simulink library "AMKMotor"  (R2015a)
settings: Solver=ode45  StartTime=0.0  StopTime=10.0  RelTol=1e-3
undefined symbols (not defined in the file): Motor
libraries: driveline x1, simulink x1
settings Model: Creator=BRIAN  LastModifiedBy=BRIAN

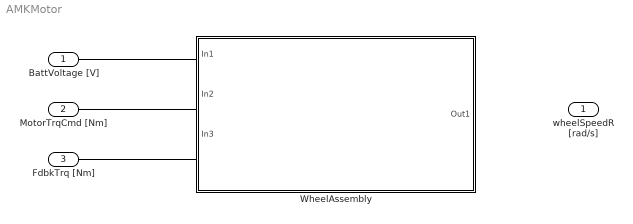
== system AMKMotor ==
  BattVoltage [V] : Inport
  MotorTrqCmd [Nm] : Inport  Port=2
  FdbkTrq [Nm] : Inport  Port=3
  WheelAssembly : Subsystem
  wheelSpeedR [rad/s] : Outport
  wires:
  BattVoltage [V]/1 -> ?
  MotorTrqCmd [Nm]/1 -> ?
  FdbkTrq [Nm]/1 -> ?
  ? -> wheelSpeedR [rad/s]/1

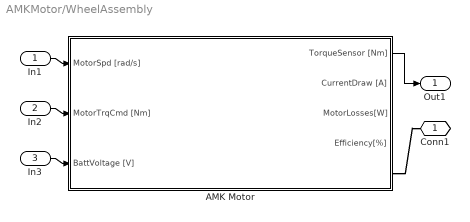
== system AMKMotor/WheelAssembly ==
  In1 : Inport
  In2 : Inport  Port=2
  In3 : Inport  Port=3
  AMK Motor : Subsystem
  Conn1 : PMIOPort  Port=1  Side=Left
  Out1 : Outport
  wires:
  In2/1 -> AMK Motor/2(MotorTrqCmd [Nm])
  In1/1 -> AMK Motor/1(MotorSpd [rad/s])
  In3/1 -> AMK Motor/3(BattVoltage [V])
  AMK Motor/1(TorqueSensor [Nm]) -> Out1/1
  connections:
  AMK Motor/RConn1 -- Conn1/RConn1

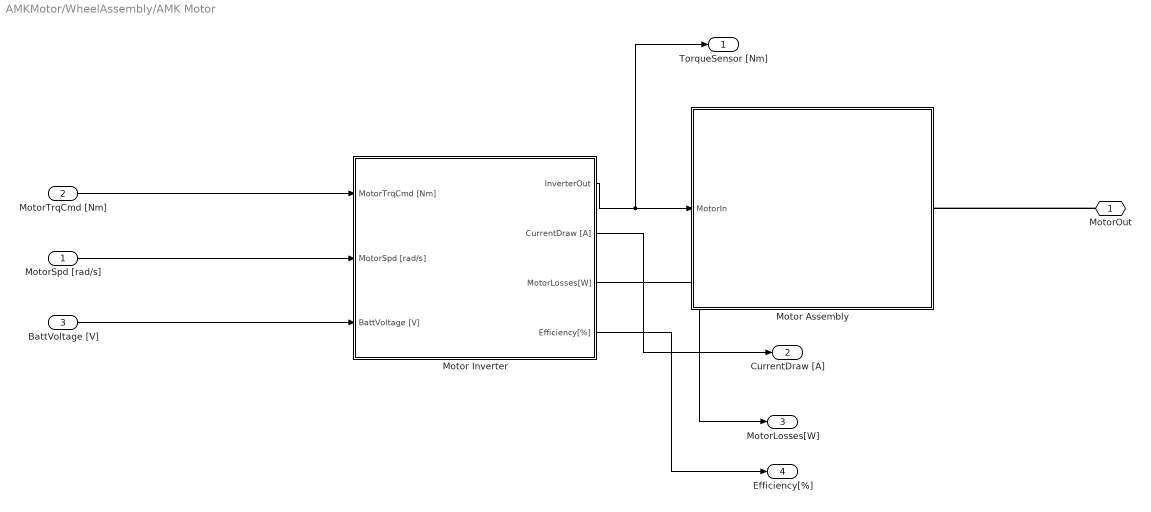
== system AMKMotor/WheelAssembly/AMK Motor ==
  MotorSpd [rad/s] : Inport
  MotorTrqCmd [Nm] : Inport  Port=2
  BattVoltage [V] : Inport  Port=3
  Motor Assembly : Subsystem
  Motor Inverter : Subsystem
  MotorOut : PMIOPort  Port=1  Side=Right
  TorqueSensor [Nm] : Outport
  CurrentDraw [A] : Outport  Port=2
  MotorLosses[W] : Outport  Port=3
  Efficiency[%] : Outport  Port=4
  wires:
  Motor Inverter/4(Efficiency[%]) -> Efficiency[%]/1
  Motor Inverter/3(MotorLosses[W]) -> MotorLosses[W]/1
  Motor Inverter/2(CurrentDraw [A]) -> CurrentDraw [A]/1
  BattVoltage [V]/1 -> Motor Inverter/3(BattVoltage [V])
  MotorSpd [rad/s]/1 -> Motor Inverter/2(MotorSpd [rad/s])
  MotorTrqCmd [Nm]/1 -> Motor Inverter/1(MotorTrqCmd [Nm])
  Motor Inverter/1(InverterOut) -> Motor Assembly/1(MotorIn), TorqueSensor [Nm]/1
  connections:
  MotorOut/RConn1 -- Motor Assembly/RConn1

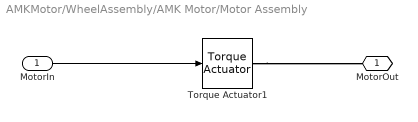
== system AMKMotor/WheelAssembly/AMK Motor/Motor Assembly ==
  MotorIn : Inport
  Torque Actuator1 : driveline/Sensors & Actuators/Torque Actuator
  MotorOut : PMIOPort  Port=1  Side=Right
  wires:
  MotorIn/1 -> Torque Actuator1/1
  connections:
  Torque Actuator1/RConn1 -- MotorOut/RConn1

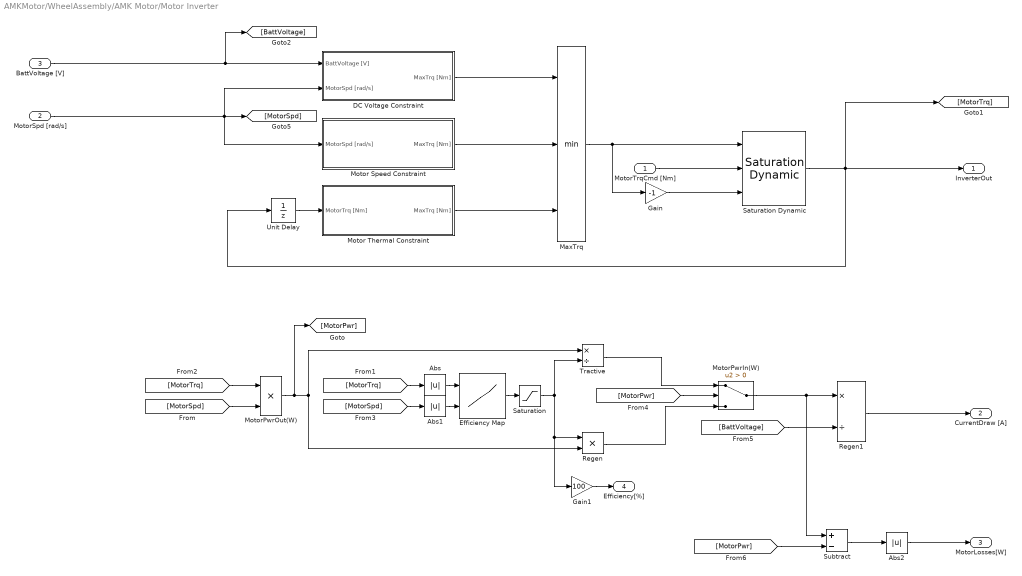
== system AMKMotor/WheelAssembly/AMK Motor/Motor Inverter ==
  MotorTrqCmd [Nm] : Inport
  MotorSpd [rad/s] : Inport  Port=2
  BattVoltage [V] : Inport  Port=3
  Abs : Abs
  Abs1 : Abs
  Abs2 : Abs
  DC Voltage Constraint : Subsystem
  Efficiency Map : Lookup_n-D  BreakpointsForDimension1=Motor.Efficiency.Trq  BreakpointsForDimension2=Motor.Efficiency.Spd  Table=Motor.Efficiency.Eff  InternalRulePriority=Speed  RndMeth=Simplest  InputSameDT=on
  Gain : Gain  Gain=-1
  Gain1 : Gain  Gain=100
  MaxTrq : MinMax  Inputs=3
  Motor Speed Constraint : Subsystem
  Motor Thermal Constraint : Subsystem
  MotorPwrIn(W) : Switch  Criteria=u2 > Threshold
  MotorPwrOut(W) : Product
  Regen : Product
  Regen1 : Product  Inputs=*/
  Saturation : Saturate  UpperLimit=1  LowerLimit=0.01
  Saturation Dynamic : simulink/Discontinuities/Saturation Dynamic  OutMin=[]  OutMax=[]  OutDataTypeStr=Inherit: Same as second input  OutDataType=fixdt(1, 16)  OutScaling=2^-10  DoSatur=off
  Subtract : Sum  Inputs=+-
  Tractive : Product  Inputs=*/
  Unit Delay : UnitDelay  SampleTime=-1
  InverterOut : Outport
  CurrentDraw [A] : Outport  Port=2
  MotorLosses[W] : Outport  Port=3
  Efficiency[%] : Outport  Port=4
  wires:
  Gain1/1 -> Efficiency[%]/1
  Abs2/1 -> MotorLosses[W]/1
  Subtract/1 -> Abs2/1
  [MotorPwr] -> Subtract/2
  Abs1/1 -> Efficiency Map/2
  Abs/1 -> Efficiency Map/1
  Saturation/1 -> Tractive/2, Regen/1, Gain1/1
  Regen1/1 -> CurrentDraw [A]/1
  [BattVoltage] -> Regen1/2
  MotorPwrIn(W)/1 -> Regen1/1, Subtract/1
  BattVoltage [V]/1 -> DC Voltage Constraint/1(BattVoltage [V]), [BattVoltage]
  Regen/1 -> MotorPwrIn(W)/3
  Tractive/1 -> MotorPwrIn(W)/1
  Efficiency Map/1 -> Saturation/1
  MotorPwrOut(W)/1 -> Tractive/1, Regen/2, [MotorPwr]
  [MotorPwr] -> MotorPwrIn(W)/2
  [MotorSpd] -> Abs1/1
  [MotorTrq] -> MotorPwrOut(W)/1
  [MotorTrq] -> Abs/1
  [MotorSpd] -> MotorPwrOut(W)/2
  MotorSpd [rad/s]/1 -> [MotorSpd], Motor Speed Constraint/1(MotorSpd [rad/s]), DC Voltage Constraint/2(MotorSpd [rad/s])
  MaxTrq/1 -> Gain/1, Saturation Dynamic/1
  Saturation Dynamic/1 -> InverterOut/1, Unit Delay/1, [MotorTrq]
  Unit Delay/1 -> Motor Thermal Constraint/1(MotorTrq [Nm])
  Gain/1 -> Saturation Dynamic/3
  Motor Thermal Constraint/1(MaxTrq [Nm]) -> MaxTrq/3
  Motor Speed Constraint/1(MaxTrq [Nm]) -> MaxTrq/2
  DC Voltage Constraint/1(MaxTrq [Nm]) -> MaxTrq/1
  MotorTrqCmd [Nm]/1 -> Saturation Dynamic/2

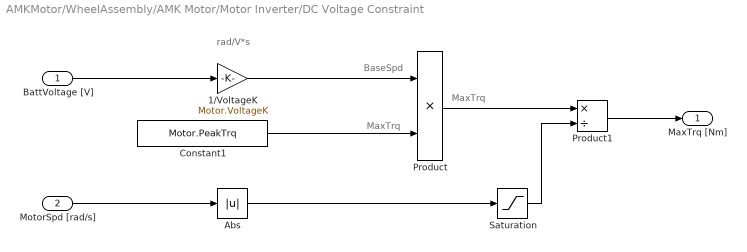
== system AMKMotor/WheelAssembly/AMK Motor/Motor Inverter/DC Voltage Constraint ==
  note: MaxTrq
  note: MaxTrq
  note: BaseSpd
  note: rad/V*s
  BattVoltage [V] : Inport
  MotorSpd [rad/s] : Inport  Port=2
  1/VoltageK : Gain  Gain=Motor.VoltageK
  Abs : Abs
  Constant1 : Constant  Value=Motor.PeakTrq
  Product : Product
  Product1 : Product  Inputs=*/
  Saturation : Saturate  UpperLimit=inf  LowerLimit=Motor.MinSpd
  MaxTrq [Nm] : Outport
  wires:
  Saturation/1 -> Product1/2
  Product/1 -> Product1/1
  BattVoltage [V]/1 -> 1/VoltageK/1
  Constant1/1 -> Product/2
  Product1/1 -> MaxTrq [Nm]/1
  MotorSpd [rad/s]/1 -> Abs/1
  1/VoltageK/1 -> Product/1
  Abs/1 -> Saturation/1

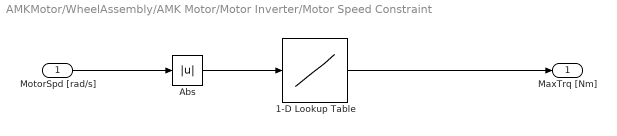
== system AMKMotor/WheelAssembly/AMK Motor/Motor Inverter/Motor Speed Constraint ==
  MotorSpd [rad/s] : Inport
  1-D Lookup Table : Lookup_n-D  NumberOfTableDimensions=1  BreakpointsForDimension1=Motor.MaxTrq.Spd  Table=Motor.MaxTrq.Trq  InternalRulePriority=Speed  RndMeth=Simplest  InputSameDT=on
  Abs : Abs
  MaxTrq [Nm] : Outport
  wires:
  MotorSpd [rad/s]/1 -> Abs/1
  1-D Lookup Table/1 -> MaxTrq [Nm]/1
  Abs/1 -> 1-D Lookup Table/1

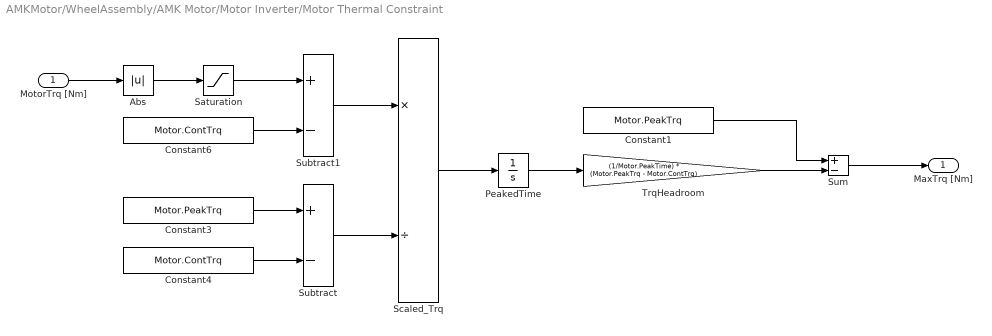
== system AMKMotor/WheelAssembly/AMK Motor/Motor Inverter/Motor Thermal Constraint ==
  MotorTrq [Nm] : Inport
  Abs : Abs
  Constant1 : Constant  Value=Motor.PeakTrq
  Constant3 : Constant  Value=Motor.PeakTrq
  Constant4 : Constant  Value=Motor.ContTrq
  Constant6 : Constant  Value=Motor.ContTrq
  PeakedTime : Integrator  LimitOutput=on  LowerSaturationLimit=0
  Saturation : Saturate  UpperLimit=Motor.PeakTrq  LowerLimit=0
  Scaled_Trq : Product  Inputs=*/
  Subtract : Sum  Inputs=+-
  Subtract1 : Sum  Inputs=+-
  Sum : Sum  Inputs=+-
  TrqHeadroom : Gain  Gain=(1/Motor.PeakTime) * (Motor.PeakTrq - Motor.ContTrq)
  MaxTrq [Nm] : Outport
  wires:
  Constant1/1 -> Sum/1
  Sum/1 -> MaxTrq [Nm]/1
  TrqHeadroom/1 -> Sum/2
  Saturation/1 -> Subtract1/1
  PeakedTime/1 -> TrqHeadroom/1
  Abs/1 -> Saturation/1
  Subtract1/1 -> Scaled_Trq/1
  Subtract/1 -> Scaled_Trq/2
  Scaled_Trq/1 -> PeakedTime/1
  Constant6/1 -> Subtract1/2
  Constant3/1 -> Subtract/1
  Constant4/1 -> Subtract/2
  MotorTrq [Nm]/1 -> Abs/1
